simulink model "Brightspace_model_simon"  (R2020b)
settings: Solver=VariableStepAuto  StartTime=0.0  StopTime=10  RelTol=1e-3
libraries: pid_lib x2
settings Model: Creator=Simon Gebraad  LastModifiedBy=Simon Gebraad

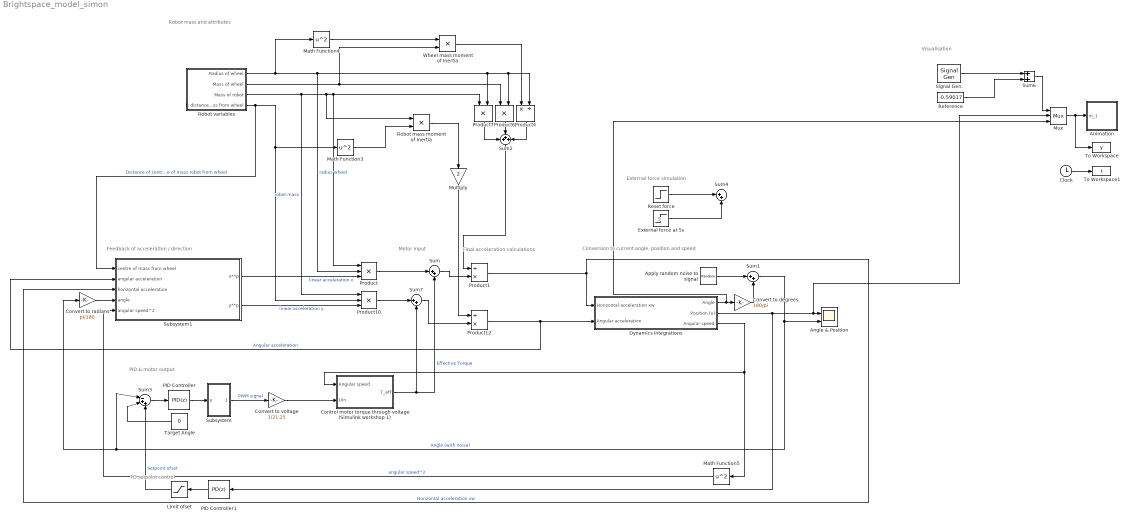
== system Brightspace_model_simon ==
  note: Visualisation
  note: External force simulation
  note: PD setpoint control
  note: 5
  note: Final acceleration
      | calculations
  note: Motor input
  note: Robot mass and attributes
  note: PID & motor output
  note: Conversion to current angle, position and speed
  note: Feedback of acceleration / direction
  Angle & Position : Scope  NumInputPorts=2
  Animation : Subsystem  mask(Pendulum plot){RefBlock=Reference}
      mask prompts: RefBlock "DC reference signal block name:"
      mask help: Pendulum plot
      mask Help: Pendulum animation function using Handle graphics.
      mask Display: plot([-10 10],[0 0],[-2 -2 2 2],[0 1 1 0],[0 3],[1 5])
  Apply random noise to signal : UniformRandomNumber  Minimum=-0.1  Maximum=0.1  SampleTime=0.01
  Clock : Clock
  Control motor torque through voltage (Simulink workshop 1) : Subsystem
  Convert to degrees : Gain  Gain=180/pi
  Convert to radians : Gain  Gain=pi/180
  Convert to voltage : Gain  Gain=1/21.25
  Dynamics integrations : Subsystem
  External force at 5s : Step  Time=5  After=10  SampleTime=0
  Limit ofset : Saturate  UpperLimit=20  LowerLimit=-20
  Math Function3 : Math  Operator=square  SaturateOnIntegerOverflow=on
  Math Function4 : Math  Operator=square  SaturateOnIntegerOverflow=on
  Math Function5 : Math  Operator=square  SaturateOnIntegerOverflow=on
  Multiply : Gain  Gain=2
  Mux : Mux  Inputs=3
  PID Controller : pid_lib/PID Controller  Controller=PID  Form=Parallel  TimeDomain=Discrete-time  UseExternalTs=off  SampleTime=-1  IntegratorMethod=Forward Euler  FilterMethod=Forward Euler  ControllerParametersSource=internal  P=23.0011804693693  I=118.837210884915  D=1.11298115094784  UseFilter=off  N=7228.80034815411  TunerSelectOption=Transfer Function Based (PID Tuner App)  InitialConditionSource=internal  InitialConditionForIntegrator=0  InitialConditionForFilter=0  DifferentiatorICPrevScaledInput=0  ExternalReset=none  TrackingMode=off  Kt=1  LimitOutput=off  SatLimitsSource=internal  UpperSaturationLimit=inf  LowerSaturationLimit=-inf  LinearizeAsGain=on  AntiWindupMode=none  Kb=1  POutMin=[]  POutMax=[]  IOutMin=[]  IOutMax=[]  DOutMin=[]  DOutMax=[]  NOutMin=[]  NOutMax=[]  SumOutMin=[]  SumOutMax=[]  SaturationOutMin=[]  SaturationOutMax=[]  PParamMin=[]  PParamMax=[]  IParamMin=[]  IParamMax=[]  DParamMin=[]  DParamMax=[]  NParamMin=[]  NParamMax=[]  KbParamMin=[]  KbParamMax=[]  KtParamMin=[]  KtParamMax=[]  KbOutMin=[]  KbOutMax=[]  KtOutMin=[]  KtOutMax=[]  IntegratorOutMin=[]  IntegratorOutMax=[]  FilterOutMin=[]  FilterOutMax=[]  SumI1OutMin=[]  SumI1OutMax=[]  SumI2OutMin=[]  SumI2OutMax=[]  SumI3OutMin=[]  SumI3OutMax=[]  SumI4OutMin=[]  SumI4OutMax=[]  SumDOutMin=[]  SumDOutMax=[]  DifferentiatorOutMin=[]  DifferentiatorOutMax=[]  FilterDiffOutCoefMin=[]  FilterDiffOutCoefMax=[]  ReciprocalOutMin=[]  ReciprocalOutMax=[]  SumDenOutMin=[]  SumDenOutMax=[]  SumNumOutMin=[]  SumNumOutMax=[]  DivideOutMin=[]  DivideOutMax=[]  UdiffTsProdOutMin=[]  UdiffTsProdOutMax=[]  NTsProdOutMin=[]  NTsProdOutMax=[]  UintegralTsProdOutMin=[]  UintegralTsProdOutMax=[]  UngainTsProdOutMin=[]  UngainTsProdOutMax=[]  IntegratorContinuousStateAttributes=''  IntegratorStateMustResolveToSignalObject=off  IntegratorRTWStateStorageClass=Auto  FilterContinuousStateAttributes=''  FilterStateMustResolveToSignalObject=off  FilterRTWStateStorageClass=Auto  ParallelPVariant=InternalParameters  IdealPVariant=Disabled  IVariant=InternalParameters  DVariant=InternalParameters  IntegratorVariant=Discrete  SatVariant=Disabled  AWVariant=Passthrough  PCopyVariant=Disabled  TRVariant=Disabled  FdbkBlocksVariant=Forward  IdealPFdbkVariant=Disabled  SatFdbkVariant=Disabled  DerivativeFilterVariant=Differentiator  NVariant=Passthrough  NCopyVariant=Disabled_SignalSpec  FilterICVariant=InternalICsDifferentiator  IntegratorICVariant=InternalICs  ExternalResetVariant=Disabled  TRSumVariant=Passthrough  SumFdbkVariant=Disabled  SumVariant=Sum_PID  TsampFilterVariant=InternalTs  TsampNgainVariant=Passthrough  TsampIntegralVariant=Passthrough  ExternalSaturationOutDataTypeStr=Inherit: Same as second input
  PID Controller1 : pid_lib/PID Controller  Controller=PD  Form=Parallel  TimeDomain=Discrete-time  UseExternalTs=off  SampleTime=-1  IntegratorMethod=Forward Euler  FilterMethod=Forward Euler  ControllerParametersSource=internal  P=0.663967610981784  I=-0.0417237045170683  D=1.53873233671338  UseFilter=off  N=7228.80034815411  TunerSelectOption=Transfer Function Based (PID Tuner App)  InitialConditionSource=internal  InitialConditionForIntegrator=0  InitialConditionForFilter=0  DifferentiatorICPrevScaledInput=0  ExternalReset=none  TrackingMode=off  Kt=1  LimitOutput=off  SatLimitsSource=internal  UpperSaturationLimit=inf  LowerSaturationLimit=-inf  LinearizeAsGain=on  AntiWindupMode=none  Kb=1  POutMin=[]  POutMax=[]  IOutMin=[]  IOutMax=[]  DOutMin=[]  DOutMax=[]  NOutMin=[]  NOutMax=[]  SumOutMin=[]  SumOutMax=[]  SaturationOutMin=[]  SaturationOutMax=[]  PParamMin=[]  PParamMax=[]  IParamMin=[]  IParamMax=[]  DParamMin=[]  DParamMax=[]  NParamMin=[]  NParamMax=[]  KbParamMin=[]  KbParamMax=[]  KtParamMin=[]  KtParamMax=[]  KbOutMin=[]  KbOutMax=[]  KtOutMin=[]  KtOutMax=[]  IntegratorOutMin=[]  IntegratorOutMax=[]  FilterOutMin=[]  FilterOutMax=[]  SumI1OutMin=[]  SumI1OutMax=[]  SumI2OutMin=[]  SumI2OutMax=[]  SumI3OutMin=[]  SumI3OutMax=[]  SumI4OutMin=[]  SumI4OutMax=[]  SumDOutMin=[]  SumDOutMax=[]  DifferentiatorOutMin=[]  DifferentiatorOutMax=[]  FilterDiffOutCoefMin=[]  FilterDiffOutCoefMax=[]  ReciprocalOutMin=[]  ReciprocalOutMax=[]  SumDenOutMin=[]  SumDenOutMax=[]  SumNumOutMin=[]  SumNumOutMax=[]  DivideOutMin=[]  DivideOutMax=[]  UdiffTsProdOutMin=[]  UdiffTsProdOutMax=[]  NTsProdOutMin=[]  NTsProdOutMax=[]  UintegralTsProdOutMin=[]  UintegralTsProdOutMax=[]  UngainTsProdOutMin=[]  UngainTsProdOutMax=[]  IntegratorContinuousStateAttributes=''  IntegratorStateMustResolveToSignalObject=off  IntegratorRTWStateStorageClass=Auto  FilterContinuousStateAttributes=''  FilterStateMustResolveToSignalObject=off  FilterRTWStateStorageClass=Auto  ParallelPVariant=InternalParameters  IdealPVariant=Disabled  IVariant=Disabled  DVariant=InternalParameters  IntegratorVariant=Disabled  SatVariant=Disabled  AWVariant=Disabled  PCopyVariant=Disabled  TRVariant=Disabled  FdbkBlocksVariant=Forward  IdealPFdbkVariant=Disabled  SatFdbkVariant=Disabled  DerivativeFilterVariant=Differentiator  NVariant=Passthrough  NCopyVariant=Disabled_SignalSpec  FilterICVariant=InternalICsDifferentiator  IntegratorICVariant=Disabled  ExternalResetVariant=Disabled  TRSumVariant=Passthrough  SumFdbkVariant=Disabled  SumVariant=Sum_PD  TsampFilterVariant=InternalTs  TsampNgainVariant=Passthrough  TsampIntegralVariant=Disabled_SignalSpec  ExternalSaturationOutDataTypeStr=Inherit: Same as second input
  Product : Product  Inputs=3
  Product1 : Product  Inputs=/*
  Product10 : Product  Inputs=3
  Product12 : Product  Inputs=/*
  Product4 : Product  Inputs=*/
  Product6 : Product
  Product7 : Product
  Reference : Constant  Value=-0.59017
  Reset force : Step  Time=5.5  After=-10  SampleTime=0
  Robot mass moment of Inertia : Product
  Robot variables : Subsystem
  Signal Gen. : SignalGenerator  WaveForm=square  Amplitude=0.000000  Frequency=0.400000  Units=rad/sec
  Subsystem : Subsystem
  Subsystem1 : Subsystem
  Sum{,1,4,7} (4 alike) : Sum  Inputs=|++
  Sum2 : Sum  Inputs=+++
  Sum3 : Sum  Inputs=|-++
  Sum6 : Sum  InputSameDT=on  SaturateOnIntegerOverflow=on  OutDataTypeStr=Inherit: Same as first input
  Target Angle : Constant  Value=0
  To Workspace : ToWorkspace  VariableName=y  SampleTime=0.1
  To Workspace1 : ToWorkspace  VariableName=t  SampleTime=0.1
  Wheel mass moment of Inertia : Product
  wires:
  Product/1 -> Sum/1
  Math Function3/1 -> Robot mass moment of Inertia/2
  Math Function4/1 -> Wheel mass moment of Inertia/1
  Wheel mass moment of Inertia/1 -> Product4/1
  Product7/1 -> Sum2/1
  Product6/1 -> Sum2/2
  Product4/1 -> Sum2/3
  Product10/1 -> Sum7/1
  Target Angle/1 -> Sum3/2
  PID Controller/1 -> Subsystem/1(y)
  Sum3/1 -> PID Controller/1
  Robot variables/2(Mass of wheel) -> Wheel mass moment of Inertia/2, Product6/1
  Robot variables/1(Radius of wheel) -> Product4/2, Product6/2, Product7/2, Product/2, Math Function4/1  "radius wheel"
  Robot variables/4(l: distance of centre of mass from wheel) -> Product10/2, Math Function3/1, Subsystem1/1(centre of mass from wheel)  "Distance of centre of mass robot from wheel"
  Robot variables/3(Mass of robot) -> Product10/1, Product/1, Product7/1, Robot mass moment of Inertia/1  "robot mass"
  Math Function5/1 -> Subsystem1/5(angular speed^2)  "angular speed^2"
  Subsystem1/1(x**p) -> Product/3  "linear acceleration x"
  Subsystem1/2(y**p) -> Product10/3  "linear acceleration y"
  Robot mass moment of Inertia/1 -> Multiply/1
  Product1/1 -> Subsystem1/3(horizontal acceleration), Dynamics integrations/1(Horizontal acceleration xw)  "Horizontal acceleration xw"
  Sum7/1 -> Product12/2
  Sum2/1 -> Product1/1
  Multiply/1 -> Product12/1
  Sum/1 -> Product1/2
  Product12/1 -> Dynamics integrations/2(Angular acceleration), Subsystem1/2(angular acceleration)  "Angular acceleration"
  Dynamics integrations/3(Angular speed) -> Control motor torque through voltage (Simulink workshop 1)/1(Angular speed), Math Function5/1
  Control motor torque through voltage (Simulink workshop 1)/1(T_eff) -> Sum/2, Sum7/2  "Effective Torque"
  Dynamics integrations/1(Angle) -> Mux/3, Convert to degrees/1
  Sum1/1 -> Angle & Position/2, Sum3/1, Convert to radians/1  "Angle (with noise)"
  Clock/1 -> To Workspace1/1
  Mux/1 -> To Workspace/1, Animation/1(in_1)
  Signal Gen./1 -> Sum6/1
  Reference/1 -> Sum6/2
  Sum6/1 -> Mux/1
  Convert to voltage/1 -> Control motor torque through voltage (Simulink workshop 1)/2(Uin)
  External force at 5s/1 -> Sum4/2
  Convert to degrees/1 -> Sum1/2
  Convert to radians/1 -> Subsystem1/4(angle)
  Reset force/1 -> Sum4/1
  Dynamics integrations/2(Position (x)) -> PID Controller1/1, Angle & Position/1, Mux/2
  PID Controller1/1 -> Limit ofset/1
  Limit ofset/1 -> Sum3/3  "Setpoint ofset"
  Subsystem/1(Out1) -> Convert to voltage/1  "PWM signal"
  Apply random noise to signal/1 -> Sum1/1

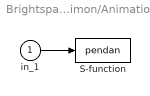
== system Brightspace_model_simon/Animation ==
  in_1 : Inport
  S-function : S-Function  FunctionName=pendan  Parameters=RefBlock  SFunctionDeploymentMode=off  EnableBusSupport=off
      settings: DeleteFcn=pendan([],[],[],'DeleteBlock');
  wires:
  in_1/1 -> S-function/1

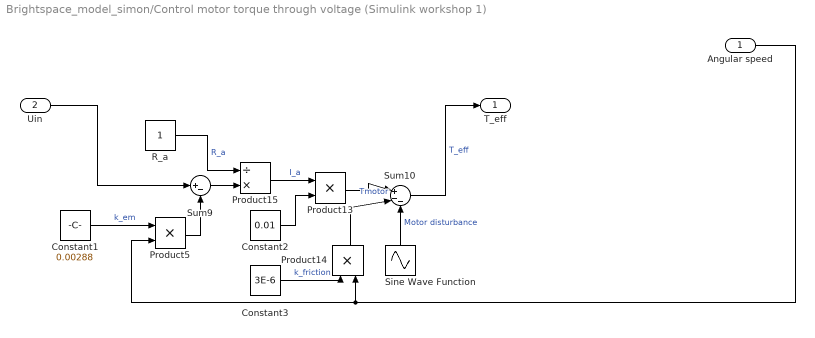
== system Brightspace_model_simon/Control motor torque through voltage (Simulink workshop 1) ==
  Angular speed : Inport
  Uin : Inport  Port=2
  Constant1 : Constant  Value=0.00288
  Constant2 : Constant  Value=0.01
  Constant3 : Constant  Value=3E-6
  Product13 : Product
  Product14 : Product
  Product15 : Product  Inputs=/*
  Product5 : Product
  R_a : Constant
  Sine Wave Function : Sin  Amplitude=0  Frequency=100  SampleTime=0
  Sum10 : Sum  Inputs=|+--
  Sum9 : Sum  Inputs=|+-
  T_eff : Outport
  wires:
  Product5/1 -> Sum9/2
  Product15/1 -> Product13/1  "I_a"
  Product14/1 -> Sum10/2
  Constant1/1 -> Product5/1  "k_em"
  Sum9/1 -> Product15/2
  Constant3/1 -> Product14/1  "k_friction"
  Constant2/1 -> Product13/2
  Angular speed/1 -> Product5/2, Product14/2
  Product13/1 -> Sum10/1  "Tmotor"
  R_a/1 -> Product15/1  "R_a"
  Uin/1 -> Sum9/1
  Sine Wave Function/1 -> Sum10/3  "Motor disturbance"
  Sum10/1 -> T_eff/1  "T_eff"

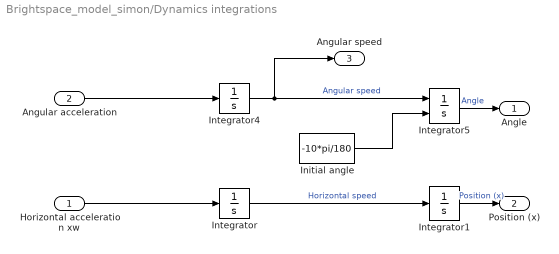
== system Brightspace_model_simon/Dynamics integrations ==
  Horizontal acceleration xw : Inport
  Angular acceleration : Inport  Port=2
  Initial angle : Constant  Value=-10*pi/180
  Integrator : Integrator
  Integrator1 : Integrator
  Integrator4 : Integrator
  Integrator5 : Integrator  InitialConditionSource=external  InitialCondition=1
  Angle : Outport
  Position (x) : Outport  Port=2
  Angular speed : Outport  Port=3
  wires:
  Horizontal acceleration xw/1 -> Integrator/1
  Initial angle/1 -> Integrator5/2
  Integrator/1 -> Integrator1/1  "Horizontal speed"
  Angular acceleration/1 -> Integrator4/1
  Integrator1/1 -> Position (x)/1  "Position (x)"
  Integrator5/1 -> Angle/1  "Angle"
  Integrator4/1 -> Integrator5/1, Angular speed/1  "Angular speed"

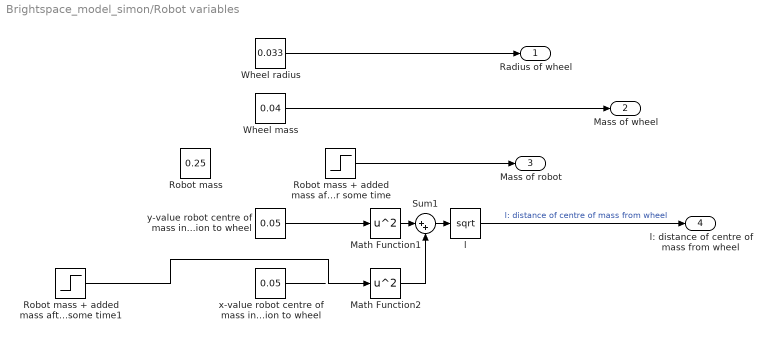
== system Brightspace_model_simon/Robot variables ==
  Math Function1 : Math  Operator=square  SaturateOnIntegerOverflow=on
  Math Function2 : Math  Operator=square  SaturateOnIntegerOverflow=on
  Robot mass : Constant  Value=0.25
  Robot mass + added mass after some time : Step  Time=2.5  Before=0.25  After=0.5  SampleTime=0
  Robot mass + added mass after some time1 : Step  Time=2.5  After=0.05  SampleTime=0
  Sum1 : Sum  Inputs=|++
  Wheel mass : Constant  Value=0.04
  Wheel radius : Constant  Value=0.033
  l : Sqrt  SaturateOnIntegerOverflow=on
  x-value robot centre of mass in relation to wheel : Constant  Value=0.05
  y-value robot centre of mass in relation to wheel : Constant  Value=0.05
  Radius of wheel : Outport
  Mass of wheel : Outport  Port=2
  Mass of robot : Outport  Port=3
  l: distance of centre of mass from wheel : Outport  Port=4
  wires:
  Wheel radius/1 -> Radius of wheel/1
  Wheel mass/1 -> Mass of wheel/1
  l/1 -> l: distance of centre of mass from wheel/1  "l: distance of centre of mass from wheel"
  Sum1/1 -> l/1
  y-value robot centre of mass in relation to wheel/1 -> Math Function1/1
  Math Function2/1 -> Sum1/2
  Math Function1/1 -> Sum1/1
  Robot mass + added mass after some time/1 -> Mass of robot/1
  Robot mass + added mass after some time1/1 -> Math Function2/1
  x-value robot centre of mass in relation to wheel/1 -> ?

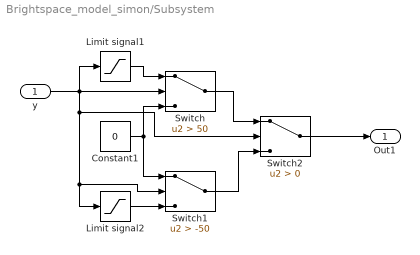
== system Brightspace_model_simon/Subsystem ==
  y : Inport
  Constant1 : Constant  Value=0
  Limit signal1 : Saturate  UpperLimit=255  LowerLimit=50
  Limit signal2 : Saturate  UpperLimit=-50  LowerLimit=-255
  Switch : Switch  Criteria=u2 > Threshold  Threshold=50
  Switch1 : Switch  Criteria=u2 > Threshold  Threshold=-50
  Switch2 : Switch  Criteria=u2 > Threshold
  Out1 : Outport
  wires:
  Limit signal1/1 -> Switch/1
  Switch/1 -> Switch2/1
  Constant1/1 -> Switch/3, Switch1/1
  Switch2/1 -> Out1/1
  y/1 -> Switch2/2, Switch1/2, Limit signal2/1, Limit signal1/1, Switch/2
  Limit signal2/1 -> Switch1/3
  Switch1/1 -> Switch2/3

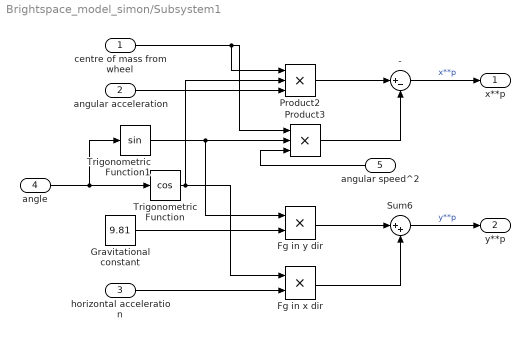
== system Brightspace_model_simon/Subsystem1 ==
  centre of mass from wheel : Inport
  angular acceleration : Inport  Port=2
  horizontal acceleration : Inport  Port=3
  angle : Inport  Port=4
  angular speed^2 : Inport  Port=5
  - : Sum  Inputs=|+-
  Fg in x dir : Product
  Fg in y dir : Product
  Gravitational constant : Constant  Value=9.81
  Product2 : Product  Inputs=3
  Product3 : Product  Inputs=3
  Sum6 : Sum  Inputs=|++
  Trigonometric Function : Trigonometry  Operator=cos
  Trigonometric Function1 : Trigonometry
  x**p : Outport
  y**p : Outport  Port=2
  wires:
  angle/1 -> Trigonometric Function1/1, Trigonometric Function/1
  angular speed^2/1 -> Product3/3
  Product2/1 -> -/1
  horizontal acceleration/1 -> Fg in x dir/2
  -/1 -> x**p/1  "x**p"
  Fg in y dir/1 -> Sum6/1
  Gravitational constant/1 -> Fg in y dir/2
  Sum6/1 -> y**p/1  "y**p"
  Product3/1 -> -/2
  angular acceleration/1 -> Product2/3
  Fg in x dir/1 -> Sum6/2
  centre of mass from wheel/1 -> Product2/1, Product3/1
  Trigonometric Function/1 -> Product2/2, Fg in x dir/1
  Trigonometric Function1/1 -> Product3/2, Fg in y dir/1
